simulink library "DYN_ATT"  (Simulink 9.0)
settings: Solver=VariableStepAuto  StartTime=0.0  StopTime=10.0  RelTol=1e-3
undefined symbols (not defined in the file): DYN_ATT_par
libraries: LIB_ROT x4
settings Model: Creator=WilTravis  LastModifiedBy=Mahal

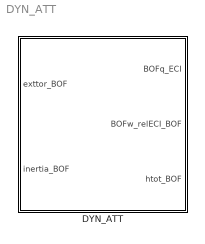
== system DYN_ATT ==
  DYN_ATT : Subsystem

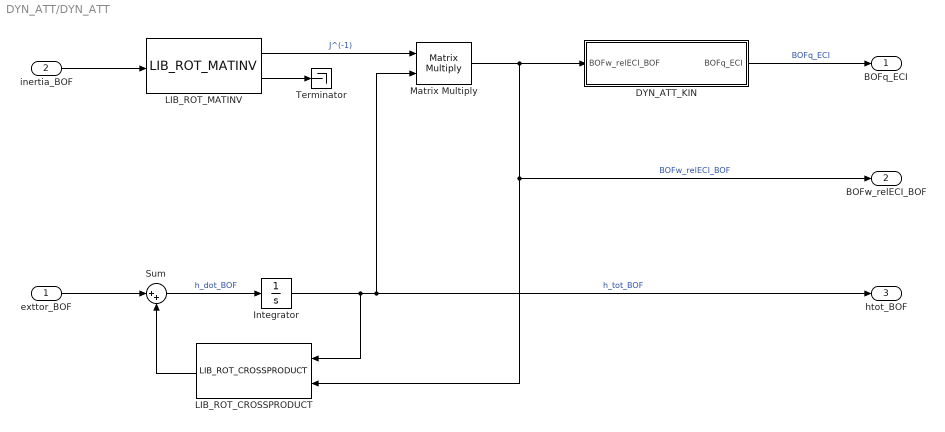
== system DYN_ATT/DYN_ATT ==
  exttor_BOF : Inport
  inertia_BOF : Inport  Port=2
  DYN_ATT_KIN : Subsystem
  Integrator : Integrator  InitialCondition=DYN_ATT_par.h_BOF_ini
  LIB_ROT_CROSSPRODUCT : LIB_ROT/LIB_ROT_CROSSPRODUCT
  "LIB_ROT_MATINV " : LIB_ROT/LIB_ROT_MATINV   tol=0
  Matrix Multiply : Product  Multiplication=Matrix(*)
  Sum : Sum  Inputs=|++
  Terminator : Terminator
  BOFq_ECI : Outport
  BOFw_relECI_BOF : Outport  Port=2
  htot_BOF : Outport  Port=3
  wires:
  Matrix Multiply/1 -> DYN_ATT_KIN/1(BOFw_relECI_BOF), LIB_ROT_CROSSPRODUCT/2, BOFw_relECI_BOF/1  "BOFw_relECI_BOF"
  Integrator/1 -> LIB_ROT_CROSSPRODUCT/1, Matrix Multiply/2, htot_BOF/1  "h_tot_BOF"
  LIB_ROT_CROSSPRODUCT/1 -> Sum/2
  Sum/1 -> Integrator/1  "h_dot_BOF"
  "LIB_ROT_MATINV "/1 -> Matrix Multiply/1  "J^(-1)"
  inertia_BOF/1 -> "LIB_ROT_MATINV "/1
  exttor_BOF/1 -> Sum/1
  DYN_ATT_KIN/1(BOFq_ECI) -> BOFq_ECI/1  "BOFq_ECI"
  "LIB_ROT_MATINV "/2 -> Terminator/1

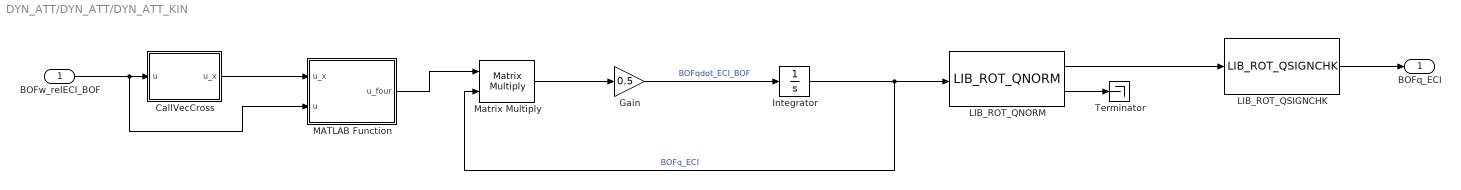
== system DYN_ATT/DYN_ATT/DYN_ATT_KIN ==
  BOFw_relECI_BOF : Inport
  CallVecCross : MATLAB Function  TreatAsAtomicUnit=on
  Gain : Gain  Gain=0.5
  Integrator : Integrator  InitialCondition=DYN_ATT_par.BOFq_ECI_ini
  LIB_ROT_QNORM : LIB_ROT/LIB_ROT_QNORM  zero_tol=0
  LIB_ROT_QSIGNCHK : LIB_ROT/LIB_ROT_QSIGNCHK  tol=0
  MATLAB Function : MATLAB Function  TreatAsAtomicUnit=on
  Matrix Multiply : Product  Multiplication=Matrix(*)
  Terminator : Terminator
  BOFq_ECI : Outport
  wires:
  Gain/1 -> Integrator/1  "BOFqdot_ECI_BOF"
  BOFw_relECI_BOF/1 -> MATLAB Function/2(u), CallVecCross/1(u)
  Integrator/1 -> LIB_ROT_QNORM/1, Matrix Multiply/2  "BOFq_ECI"
  Matrix Multiply/1 -> Gain/1
  LIB_ROT_QSIGNCHK/1 -> BOFq_ECI/1
  CallVecCross/1(u_x) -> MATLAB Function/1(u_x)
  LIB_ROT_QNORM/1 -> LIB_ROT_QSIGNCHK/1
  LIB_ROT_QNORM/2 -> Terminator/1
  MATLAB Function/1(u_four) -> Matrix Multiply/1

== matlab function DYN_ATT/DYN_ATT_KIN/MATLAB Function ==
  data: u_x input double; u input double; u_four output double
function u_four = fourXfour(u_x,u)

u_four = [-u_x, u; 
          -u', 0];

end

== matlab function DYN_ATT/DYN_ATT_KIN/CallVecCross ==
  data: u input double; u_x output double
function u_x = CallVecCross(u)

u_x = VecCross(u);

end
